simulink model "ballbeam_sim"  (Simulink 8.3)
settings: Solver=ode45  StartTime=0.0  StopTime=100  RelTol=1e-3
undefined symbols (not defined in the file or in its folder): AP, drawBallBeam, P
libraries: cstblocks x2
settings Model: Creator=beard  LastModifiedBy=jhl48
settings OptimizationCC: ExpressionDepthLimit=2147483647  InitFltsAndDblsToZero=on
settings DebuggingCC: FcnCallInpInsideContextMsg=UseLocalSettings

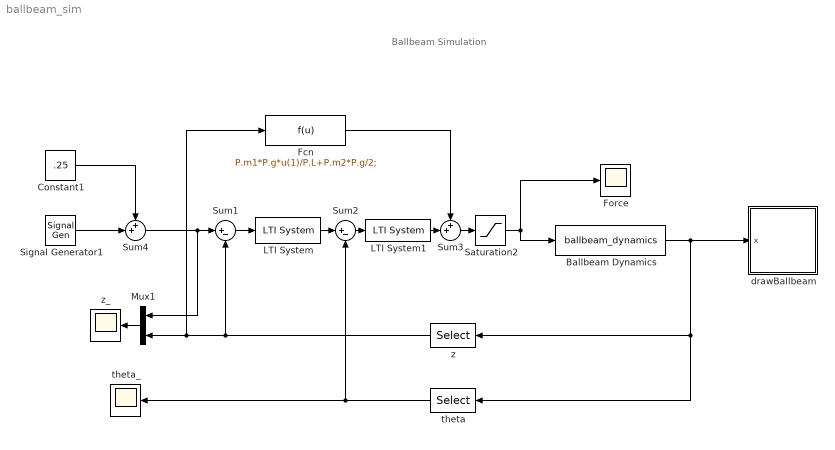
== system ballbeam_sim ==
  note: Ballbeam Simulation
  Ballbeam Dynamics : S-Function  FunctionName=ballbeam_dynamics  Parameters=AP  EnableBusSupport=off
  Constant1 : Constant  Value=.25
  Fcn : Fcn  Expr=P.m1*P.g*u(1)/P.L+P.m2*P.g/2;
  Force : Scope
      settings: TimeRange=100  YMin=9  YMax=12.25
  LTI System : cstblocks/LTI System  sys=c_outer  IC=[]
  LTI System1 : cstblocks/LTI System  sys=c_inner  IC=[]
  Mux1 : Mux  Inputs=2
  Saturation2 : Saturate  UpperLimit=AP.F_max  LowerLimit=-AP.F_max
  Signal Generator1 : SignalGenerator  WaveForm=square  Amplitude=.125  Frequency=.02
  Sum1 : Sum  Inputs=|+-
  Sum2 : Sum  Inputs=|+-
  Sum3 : Sum  Inputs=++|
  Sum4 : Sum  Inputs=++|
  drawBallbeam : Subsystem
      mask init:
      | % drawing parameters
      | L = 0.5;
      | R = .03;
      mask Display: image(imread('tv.jpg'))
  theta : Selector  InputPortWidth=2  Indices=[1]
  theta_ : Scope
      settings: TimeRange=100  YMin=-1.2e-07  YMax=-2e-08
  z : Selector  InputPortWidth=2  Indices=[2]
  z_ : Scope
      settings: TimeRange=100  YMin=0.05  YMax=0.425  SaveName=ScopeData2
  wires:
  Ballbeam Dynamics/1 -> theta/1, z/1, drawBallbeam/1(x)
  Mux1/1 -> z_/1
  Saturation2/1 -> Ballbeam Dynamics/1, Force/1
  z/1 -> Sum1/2, Fcn/1, Mux1/2
  theta/1 -> Sum2/2, theta_/1
  Sum4/1 -> Sum1/1, Mux1/1
  Sum1/1 -> LTI System/1
  LTI System/1 -> Sum2/1
  Sum2/1 -> LTI System1/1
  Fcn/1 -> Sum3/1
  Sum3/1 -> Saturation2/1
  LTI System1/1 -> Sum3/2
  Signal Generator1/1 -> Sum4/2
  Constant1/1 -> Sum4/1

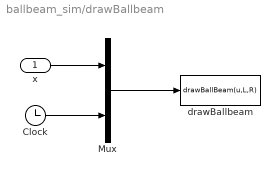
== system ballbeam_sim/drawBallbeam ==
  x : Inport
  Clock : Clock
  Mux : Mux  Inputs=2
  drawBallbeam : MATLABFcn  MATLABFcn=drawBallBeam(u,L,R)  OutputDimensions=0  SampleTime=0.01
  wires:
  Mux/1 -> drawBallbeam/1
  x/1 -> Mux/1
  Clock/1 -> Mux/2
